simulink model "TestLinearisedModel"  (R2018b)
settings: Solver=VariableStepAuto  StartTime=0.0  StopTime=30  RelTol=1e-3
undefined symbols (not defined in the file): K, sys
libraries: simulink_extras x1
settings Model: Creator=jban039  LastModifiedBy=jban039

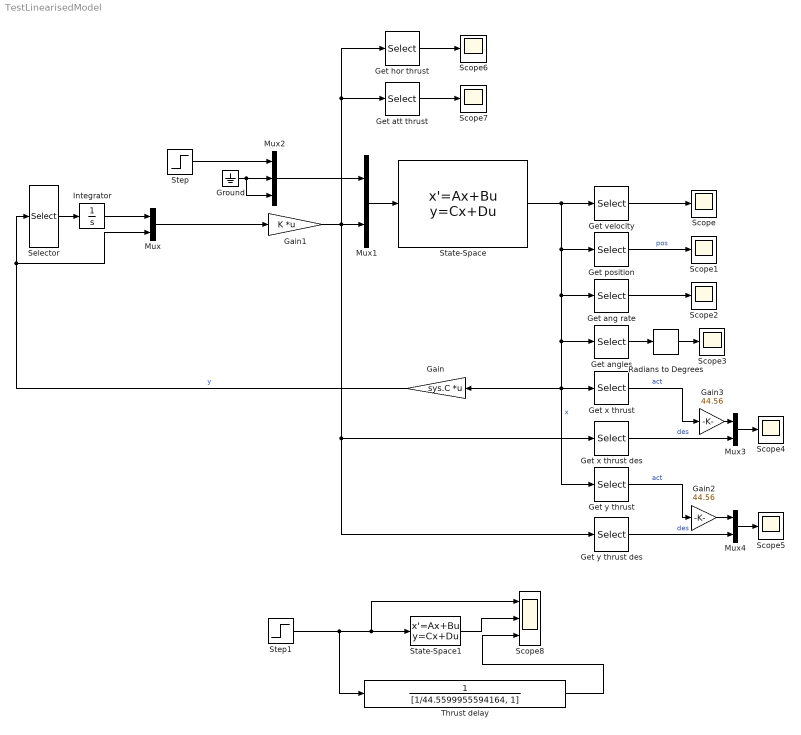
== system TestLinearisedModel ==
  Gain : Gain  Gain=sys.C  Multiplication=Matrix(K*u)
  Gain1 : Gain  Gain=K  Multiplication=Matrix(K*u)
  Gain2 : Gain  Gain=44.56
  Gain3 : Gain  Gain=44.56
  Get ang rate : Selector  InputPortWidth=12  IndexOptions=Index vector (dialog)  Indices=[7:8]  OutputSizes=1
  Get angles : Selector  InputPortWidth=12  IndexOptions=Index vector (dialog)  Indices=[9:10]  OutputSizes=1
  Get att thrust : Selector  InputPortWidth=5  IndexOptions=Index vector (dialog)  Indices=[3:5]  OutputSizes=1
  Get hor thrust : Selector  InputPortWidth=5  IndexOptions=Index vector (dialog)  Indices=[1:2]  OutputSizes=1
  Get position : Selector  InputPortWidth=12  IndexOptions=Index vector (dialog)  Indices=[4:6]  OutputSizes=1
  Get velocity : Selector  InputPortWidth=12  IndexOptions=Index vector (dialog)  Indices=[1:3]  OutputSizes=1
  Get x thrust : Selector  InputPortWidth=12  IndexOptions=Index vector (dialog)  Indices=[11]  OutputSizes=1
  Get x thrust des : Selector  InputPortWidth=5  IndexOptions=Index vector (dialog)  Indices=[1]  OutputSizes=1
  Get y thrust : Selector  InputPortWidth=12  IndexOptions=Index vector (dialog)  Indices=[12]  OutputSizes=1
  Get y thrust des : Selector  InputPortWidth=5  IndexOptions=Index vector (dialog)  Indices=[2]  OutputSizes=1
  Ground : Ground
  Integrator : Integrator
  Mux{,1,3..4} (4 alike) : Mux  Inputs=2
  Mux2 : Mux  Inputs=3
  Radians to Degrees : simulink_extras/Transformations/Radians to Degrees
  Scope{,1..7} (8 alike) : Scope
  Scope8 : Scope  NumInputPorts=3
  Selector : Selector  InputPortWidth=6  IndexOptions=Index vector (dialog)  Indices=[4:6]  OutputSizes=1
  State-Space : StateSpace  A=sys.A  B=sys.B  C=eye(size(sys.A))  D=zeros(size(sys.A,1),size(sys.B,2))  InitialCondition=0
  State-Space1 : StateSpace  A=-44.56  B=44.56  D=0  InitialCondition=0
  Step : Step  After=2  SampleTime=0
  Step1 : Step  SampleTime=0
  Thrust delay : TransferFcn  Denominator=|  ContinuousStateAttributes='Th_x'
      | [1/44.5599955594164,
      | 1]
  wires:
  State-Space/1 -> Get velocity/1, Get y thrust/1, Gain/1, Get x thrust/1, Get angles/1, Get ang rate/1, Get position/1  "x"
  Gain/1 -> Mux/2, Selector/1  "y"
  Gain1/1 -> Get hor thrust/1, Get att thrust/1, Get y thrust des/1, Get x thrust des/1, Mux1/2
  Selector/1 -> Integrator/1
  Integrator/1 -> Mux/1
  Mux/1 -> Gain1/1
  Mux1/1 -> State-Space/1
  Mux2/1 -> Mux1/1
  Step/1 -> Mux2/1
  Ground/1 -> Mux2/3, Mux2/2
  Get velocity/1 -> Scope/1
  Get ang rate/1 -> Scope2/1
  Get angles/1 -> Radians to Degrees/1
  Get x thrust/1 -> Gain3/1  "act"
  Get x thrust des/1 -> Mux3/2  "des"
  Mux3/1 -> Scope4/1
  Mux4/1 -> Scope5/1
  Get y thrust des/1 -> Mux4/2  "des"
  Get y thrust/1 -> Gain2/1  "act"
  Radians to Degrees/1 -> Scope3/1
  Get hor thrust/1 -> Scope6/1
  Get att thrust/1 -> Scope7/1
  Step1/1 -> Thrust delay/1, Scope8/1, State-Space1/1
  State-Space1/1 -> Scope8/2
  Thrust delay/1 -> Scope8/3
  Gain2/1 -> Mux4/1
  Gain3/1 -> Mux3/1
  Get position/1 -> Scope1/1  "pos"
